simulink model "Model_2a"  (R2015b)
settings: Solver=ode45  StartTime=0.0  StopTime=10  MaxStep=1e-3  RelTol=1e-3
undefined symbols (not defined in the file): g0, K, K1, p1
settings Model: Creator=s3blanch  LastModifiedBy=s3blanch
settings DataIOCC: SaveFormat=StructureWithTime
settings HardwareCC: ProdWordSize=32  ProdHWDeviceType=Specified

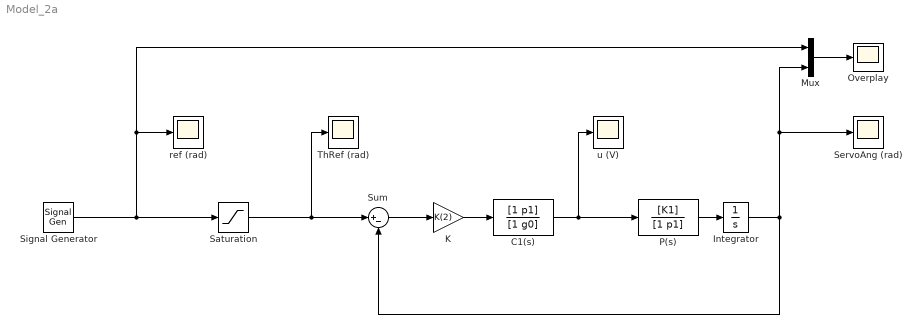
== system Model_2a ==
  C1(s) : TransferFcn  Numerator=[1 p1]  Denominator=[1 g0]
  Integrator : Integrator
  K : Gain  Gain=K(2)
  Mux : Mux  Inputs=2
  Overplay : Scope
  P(s) : TransferFcn  Numerator=[K1]  Denominator=[1 p1]
  Saturation : Saturate  UpperLimit=0.7  LowerLimit=-0.7
  ServoAng (rad) : Scope
  Signal Generator : SignalGenerator  WaveForm=square  Amplitude=-0.5  Frequency=0.2
  Sum : Sum  Inputs=|+-
  ThRef (rad) : Scope
  ref (rad) : Scope
  u (V) : Scope
  wires:
  P(s)/1 -> Integrator/1
  Sum/1 -> K/1
  Integrator/1 -> Sum/2, Mux/2, ServoAng (rad)/1
  Saturation/1 -> Sum/1, ThRef (rad)/1
  K/1 -> C1(s)/1
  C1(s)/1 -> P(s)/1, u (V)/1
  Signal Generator/1 -> Saturation/1, ref (rad)/1, Mux/1
  Mux/1 -> Overplay/1
